simulink model "eval_longitudinal_ctrl_accel"  (R2013b)
settings: Solver=FixedStepDiscrete  StartTime=0.0  StopTime=inf  RelTol=1e-3
libraries: SCANeR_API x2
settings Model: Creator=sphilippe  LastModifiedBy=sphilippe
settings RTWCC: SystemTargetFile=grt_scanerapi.tlc  TemplateMakefile=grt_scanerapi_vc.tmf  Description=SCANeR API Real-Time Target  ProcessScript=grt_scanerapi_make_rtw_hook
settings STFCustomTargetCC: GeneratePreprocessorConditionals=Disable all  MatFileLogging=on  SystemTargetFile=grt_scanerapi.tlc
settings GRTTargetCC: ParMdlRefBuildCompliant=off  CompOptLevelCompliant=off  ConcurrentExecutionCompliant=off  CombineOutputUpdateFcns=off  GRTInterface=on

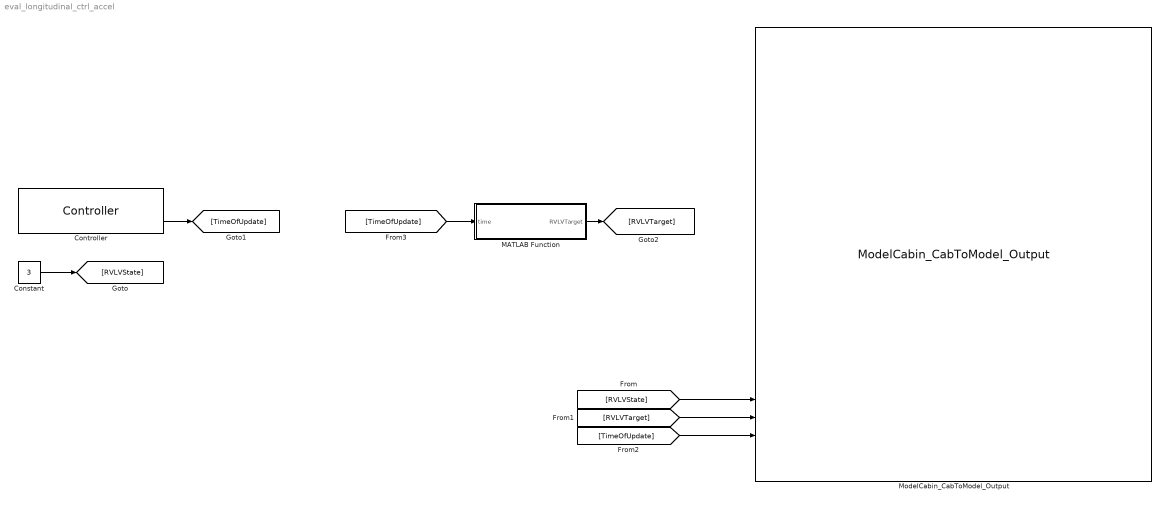
== system eval_longitudinal_ctrl_accel ==
  Constant : Constant  Value=3
  Controller : SCANeR_API/Controller  Priority=1  Config='EVAL_LONGI_CTRL_16'  ProcName='LONGI_SMLNK'  Frequency=100  NetworkOutputFrequency=10  IsSynchronized=off
  MATLAB Function : MATLAB Function  TreatAsAtomicUnit=on
  ModelCabin_CabToModel_Output : SCANeR_API/SHM outputs/ModelCabin/ModelCabin_CabToModel_Output  Priority=2  shmId=0
  wires:
  Constant/1 -> [RVLVState]
  [RVLVState] -> ModelCabin_CabToModel_Output/21
  [RVLVTarget] -> ModelCabin_CabToModel_Output/22
  Controller/2 -> [TimeOfUpdate]
  [TimeOfUpdate] -> ModelCabin_CabToModel_Output/23
  [TimeOfUpdate] -> MATLAB Function/1(time)
  MATLAB Function/1(RVLVTarget) -> [RVLVTarget]

== matlab function eval_longitudinal_ctrl_accel/MATLAB Function ==
  data: time input; RVLVTarget output
function RVLVTarget = fcn(time)
%#codegen

if (time < 10)
    RVLVTarget = 1.1;
else
    if (time < 20)
        RVLVTarget = 0;
    else
        RVLVTarget = -1.1;
    end
end
